simulink model "GSA_System"  (Simulink 7.6)
settings: Solver=ode3  StartTime=0.0  StopTime=10  FixedStep=0.001  RelTol=1e-3
undefined symbols (not defined in the file or in its folder): GSAmain
libraries: simulink x2, cstblocks x2
settings Model: Creator=hi  LastModifiedBy=admin
settings DebuggingCC: AlgebraicLoopMsg=none  ArtificialAlgebraicLoopMsg=none

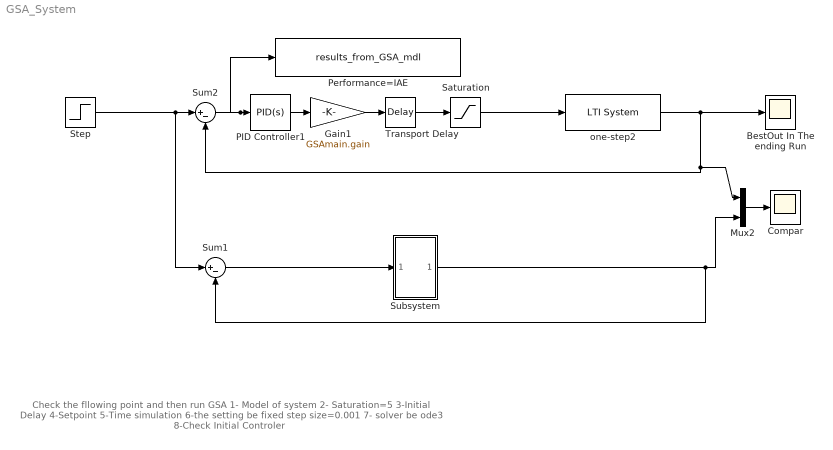
== system GSA_System ==
  note: Check the fllowing point and then run GSA
      | 1- Model of system
      | 2- Saturation=5
      | 3-Initial Delay
      | 4-Setpoint
      | 5-Time simulation
      | 6-the setting be fixed step size=0.001
      | 7- solver be ode3
      | 8-Check Initial Controler
  BestOut In The ending Run : Scope
      settings: TimeRange=1  YMin=327.5  YMax=375  SaveName=BestOutput
  "Compar " : Scope
      settings: TimeRange=1  YMin=199.725  YMax=200.025
  Gain1 : Gain  Gain=GSAmain.gain  SampleTime=0.001
  Mux2 : Mux  Inputs=2
  PID Controller1 : simulink/Continuous/PID Controller  DialogController=pidpack.PIDConfig.pidDDGCreate  DialogControllerArgs=DataTag0  SystemSampleTime=-1  Controller=PID  TimeDomain=Continuous-time  SampleTime=1  IntegratorMethod=Forward Euler  FilterMethod=Forward Euler  Form=Parallel  P=GSAmain.KP  I=GSAmain.KI  D=GSAmain.KD  N=100  InitialConditionSource=internal  InitialConditionForIntegrator=0  InitialConditionForFilter=0  ExternalReset=none  LimitOutput=off  UpperSaturationLimit=inf  LowerSaturationLimit=-inf  LinearizeAsGain=off  AntiWindupMode=none  Kb=1  TrackingMode=off  Kt=1  PParamMin=[]  PParamMax=[]  IParamMin=[]  IParamMax=[]  DParamMin=[]  DParamMax=[]  NParamMin=[]  NParamMax=[]  KbParamMin=[]  KbParamMax=[]  KtParamMin=[]  KtParamMax=[]  POutMin=[]  POutMax=[]  IOutMin=[]  IOutMax=[]  DOutMin=[]  DOutMax=[]  NOutMin=[]  NOutMax=[]  KbOutMin=[]  KbOutMax=[]  KtOutMin=[]  KtOutMax=[]  IntegratorOutMin=[]  IntegratorOutMax=[]  FilterOutMin=[]  FilterOutMax=[]  SumOutMin=[]  SumOutMax=[]  SumI1OutMin=[]  SumI1OutMax=[]  SumI2OutMin=[]  SumI2OutMax=[]  SumI3OutMin=[]  SumI3OutMax=[]  SumDOutMin=[]  SumDOutMax=[]  SaturationOutMin=[]  SaturationOutMax=[]  IntegratorContinuousStateAttributes=''  IntegratorStateMustResolveToSignalObject=off  IntegratorRTWStateStorageClass=Auto  FilterContinuousStateAttributes=''  FilterStateMustResolveToSignalObject=off  FilterRTWStateStorageClass=Auto
  Performance=IAE : ToWorkspace  VariableName=results_from_GSA_mdl  SampleTime=0.001  SaveFormat=Structure With Time
  Saturation : Saturate  UpperLimit=5  LowerLimit=-5  SampleTime=0.001
  Step : Step  Time=0  After=100  SampleTime=0.001
  Subsystem : Subsystem
  Sum1 : Sum  Inputs=|+-  SampleTime=0.001
  Sum2 : Sum  Inputs=|+-  SampleTime=0.001
  Transport Delay : TransportDelay  DelayTime=GSAmain.delay+0.04
  one-step2 : cstblocks/LTI System  SystemSampleTime=-1  sys=tf(70,[0.17 1])  IC=[]
  wires:
  Step/1 -> Sum2/1, Sum1/1
  Sum2/1 -> PID Controller1/1, Performance=IAE/1
  PID Controller1/1 -> Gain1/1
  Gain1/1 -> Transport Delay/1
  Transport Delay/1 -> Saturation/1
  one-step2/1 -> Sum2/2, Mux2/1, BestOut In The ending Run/1
  Sum1/1 -> Subsystem/1(In1)
  Subsystem/1(Out1) -> Mux2/2, Sum1/2
  Saturation/1 -> one-step2/1
  Mux2/1 -> "Compar "/1

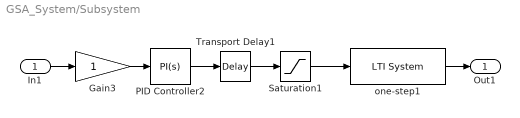
== system GSA_System/Subsystem ==
  In1 : Inport
  Gain3 : Gain  SampleTime=.001
  PID Controller2 : simulink/Continuous/PID Controller  DialogController=pidpack.PIDConfig.pidDDGCreate  DialogControllerArgs=DataTag1  SystemSampleTime=-1  Controller=PI  TimeDomain=Continuous-time  SampleTime=1  IntegratorMethod=Forward Euler  FilterMethod=Forward Euler  Form=Parallel  P=0.44  I=0.22  D=GSAmain.KD  N=100  InitialConditionSource=internal  InitialConditionForIntegrator=0  InitialConditionForFilter=0  ExternalReset=none  LimitOutput=off  UpperSaturationLimit=inf  LowerSaturationLimit=-inf  LinearizeAsGain=off  AntiWindupMode=none  Kb=1  TrackingMode=off  Kt=1  PParamMin=[]  PParamMax=[]  IParamMin=[]  IParamMax=[]  DParamMin=[]  DParamMax=[]  NParamMin=[]  NParamMax=[]  KbParamMin=[]  KbParamMax=[]  KtParamMin=[]  KtParamMax=[]  POutMin=[]  POutMax=[]  IOutMin=[]  IOutMax=[]  DOutMin=[]  DOutMax=[]  NOutMin=[]  NOutMax=[]  KbOutMin=[]  KbOutMax=[]  KtOutMin=[]  KtOutMax=[]  IntegratorOutMin=[]  IntegratorOutMax=[]  FilterOutMin=[]  FilterOutMax=[]  SumOutMin=[]  SumOutMax=[]  SumI1OutMin=[]  SumI1OutMax=[]  SumI2OutMin=[]  SumI2OutMax=[]  SumI3OutMin=[]  SumI3OutMax=[]  SumDOutMin=[]  SumDOutMax=[]  SaturationOutMin=[]  SaturationOutMax=[]  IntegratorContinuousStateAttributes=''  IntegratorStateMustResolveToSignalObject=off  IntegratorRTWStateStorageClass=Auto  FilterContinuousStateAttributes=''  FilterStateMustResolveToSignalObject=off  FilterRTWStateStorageClass=Auto
  Saturation1 : Saturate  UpperLimit=5  LowerLimit=-5  SampleTime=0.001
  Transport Delay1 : TransportDelay  DelayTime=GSAmain.delay+0.02
  one-step1 : cstblocks/LTI System  SystemSampleTime=-1  sys=tf(70,[0.17 1])  IC=[]
  Out1 : Outport
  wires:
  Gain3/1 -> PID Controller2/1
  PID Controller2/1 -> Transport Delay1/1
  Transport Delay1/1 -> Saturation1/1
  Saturation1/1 -> one-step1/1
  In1/1 -> Gain3/1
  one-step1/1 -> Out1/1
